simulink model "ART"  (Simulink 7.8)
settings: Solver=ode2  StartTime=0.0  StopTime=5  FixedStep=T  RelTol=1e-3
InitFcn:
  | mag1 = 48144;
  | mag2 = 45845;
  | trise = 0.02;
  | tfall  = 0.04;
  | [num_syn den_syn] = filter_coef(mag1, mag2, trise, tfall,T)
undefined symbols (not defined in the file or in its folder): den_syn, num_syn, SIZE_MU_11, SIZE_MU_3, T
libraries: simulink x3
settings Model: Creator=eric  LastModifiedBy=eric

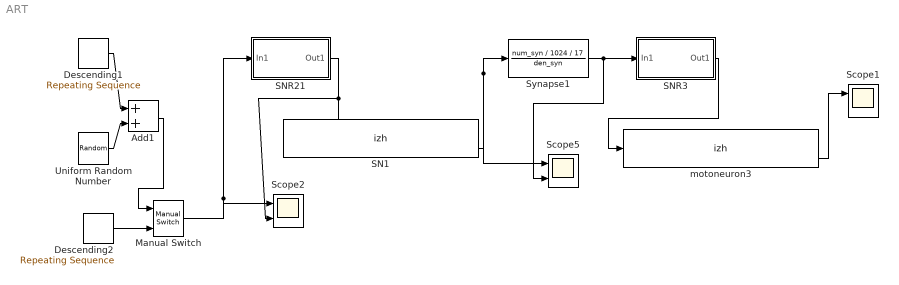
== system ART ==
  Add1 : Sum
  Descending1 : simulink/Sources/Repeating Sequence  rep_seq_t=[0 1.1 3.1 6.8 9.5 10 ]  rep_seq_y=[0 0 20 20 0 0]*1
  Descending2 : simulink/Sources/Repeating Sequence  rep_seq_t=[0 0.5 1]  rep_seq_y=[0 200 200]*0
  Manual Switch : simulink/Signal Routing/Manual Switch  sw=1  action=0  varsize=off
  SN1 : S-Function  FunctionName=izh  Parameters=[0.02 0.2 -65.0 6.0 30.0 SIZE_MU_11] [-70.0 -14.0]  EnableBusSupport=off
      mask Display:
      | port_label('input', 1, 'syn curr');
      | port_label('output', 1, 'action potential');
      | port_label('output', 2, 'spike');
      | disp('Izhi Neuron \n(S-Function)')
  SNR21 : Subsystem
  SNR3 : Subsystem
  Scope1 : Scope  NumInputPorts=2
      settings: TimeRange=10  YMin=0~-5  YMax=37.5~5  SaveName=total_force1  DataFormat=Structure
  Scope2 : Scope  NumInputPorts=2
      settings: TimeRange=10  YMin=0~-5  YMax=37.5~5  SaveName=total_force2  DataFormat=Structure
  Scope5 : Scope  NumInputPorts=2
      settings: TimeRange=10  YMin=0~-5  YMax=37.5~5  SaveName=total_force  DataFormat=Structure
  Synapse1 : DiscreteTransferFcn  Numerator=num_syn / 1024 / 17  Denominator=den_syn  SampleTime=T
  Uniform Random Number : UniformRandomNumber  Minimum=-6  Maximum=0  SampleTime=T
  motoneuron3 : S-Function  FunctionName=izh  Parameters=[0.02 0.2 -65.0 6.0 30.0 SIZE_MU_3] [-70.0 -14.0]  EnableBusSupport=off
      mask Display:
      | port_label('input', 1, 'syn curr');
      | port_label('output', 1, 'action potential');
      | port_label('output', 2, 'spike');
      | disp('Izhi Neuron \n(S-Function)')
  wires:
  SNR21/1(Out1) -> SN1/1, Scope2/2
  Add1/1 -> Manual Switch/1
  Uniform Random Number/1 -> Add1/2
  Descending2/1 -> Manual Switch/2
  Descending1/1 -> Add1/1
  Manual Switch/1 -> SNR21/1(In1), Scope2/1
  SN1/2 -> Synapse1/1, Scope5/1
  Synapse1/1 -> SNR3/1(In1), Scope5/2
  SNR3/1(Out1) -> motoneuron3/1
  motoneuron3/2 -> Scope1/1

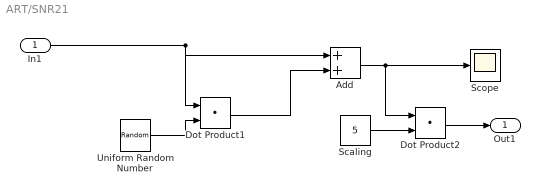
== system ART/SNR21 ==
  In1 : Inport
  Add : Sum
  Dot Product1 : DotProduct  InputSameDT=on  OutDataTypeStr=Inherit: Inherit via internal rule
  Dot Product2 : DotProduct  InputSameDT=on  OutDataTypeStr=Inherit: Inherit via internal rule
  Scaling : Constant  Value=5
  Scope : Scope
  Uniform Random Number : UniformRandomNumber  Minimum=-0.3  Maximum=0.3  SampleTime=T
  Out1 : Outport
  wires:
  Uniform Random Number/1 -> Dot Product1/2
  In1/1 -> Dot Product1/1, Add/1
  Dot Product1/1 -> Add/2
  Add/1 -> Scope/1, Dot Product2/1
  Dot Product2/1 -> Out1/1
  Scaling/1 -> Dot Product2/2

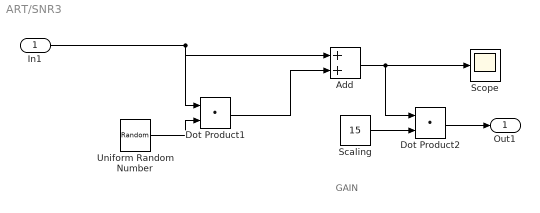
== system ART/SNR3 ==
  note: GAIN
  In1 : Inport
  Add : Sum
  Dot Product1 : DotProduct  InputSameDT=on  OutDataTypeStr=Inherit: Inherit via internal rule
  Dot Product2 : DotProduct  InputSameDT=on  OutDataTypeStr=Inherit: Inherit via internal rule
  Scaling : Constant  Value=15
  Scope : Scope
  Uniform Random Number : UniformRandomNumber  Minimum=-0.3  Maximum=0.3  SampleTime=T
  Out1 : Outport
  wires:
  Scaling/1 -> Dot Product2/2
  Dot Product2/1 -> Out1/1
  Add/1 -> Dot Product2/1, Scope/1
  Dot Product1/1 -> Add/2
  In1/1 -> Add/1, Dot Product1/1
  Uniform Random Number/1 -> Dot Product1/2
